simulink model "Pacemaker_Simulink"  (R2023a)
settings: Solver=FixedStepAuto  StartTime=0.0  StopTime=10.0  FixedStep=1e-3  RelTol=1e-3  EnableMultiTasking=on
undefined symbols (not defined in the file): A0, A1, D0, D1, D10, D11, D12, D13, D2, D3, D4, D5, D6, D7, D8, D9, magnitude, PTA0, PTA1, PTA2, PTB2, PTB23, PTB3, PTB9, PTC16, PTC17, PTC2, PTC3, PTC4, PTD0, PTD1, PTD2, PTD3
libraries: simulink x26, frdmk64flib x20, etargetslib x2, dspstat3 x1
settings Model: ExtModeTrigDuration=5  Creator=anshm  LastModifiedBy=anshm
settings OptimizationCC: EnhancedBackFolding=on  PassReuseOutputArgsAs=Individual arguments  ZeroExternalMemoryAtStartup=off  ZeroInternalMemoryAtStartup=off  MaxStackSize=64  OptimizeBlockOrder=speed  DifferentSizesBufferReuse=on  OptimizationCustomize=off  EfficientTunableParamExpr=on
settings DebuggingCC: ParameterTunabilityLossMsg=error
settings HardwareCC: ProdBitPerPointer=32  ProdBitPerSizeT=32  ProdBitPerPtrDiffT=32  ProdLargestAtomicInteger=Long  ProdLargestAtomicFloat=Double  ProdWordSize=32  ProdHWDeviceType=ARM Compatible->ARM Cortex
settings SFSimCC: MATLABDynamicMemAlloc=off
settings RTWCC: Description=Embedded Coder  SystemTargetFile=ert.tlc  HardwareBoard=NXP FRDM-K64F  TLCOptions="-aInlineSetEventsForThisBaseRateFcn=TLC_FALSE -aSuppressMultiTaskScheduler=TLC_FALSE  -aRateBasedStepFcn=0"  TemplateMakefile=ert_default_tmf  Toolchain=GNU Tools for ARM Embedded Processors
settings CodeAppCC: ForceParamTrailComments=on  IgnoreCustomStorageClasses=off  OperatorAnnotations=on  SimulinkDataObjDesc=on  SFDataObjDesc=on  InsertBlockDesc=on
settings ERTTargetCC: ExtModeTransport=4  ExtModeMexFile=sendToCommService

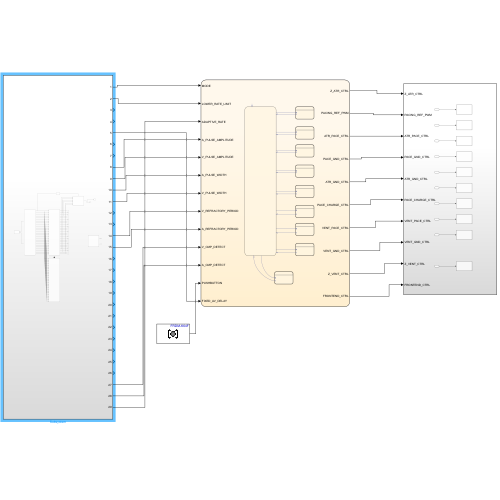
[thumbnail: Simulink's stored preview of the top-level diagram]
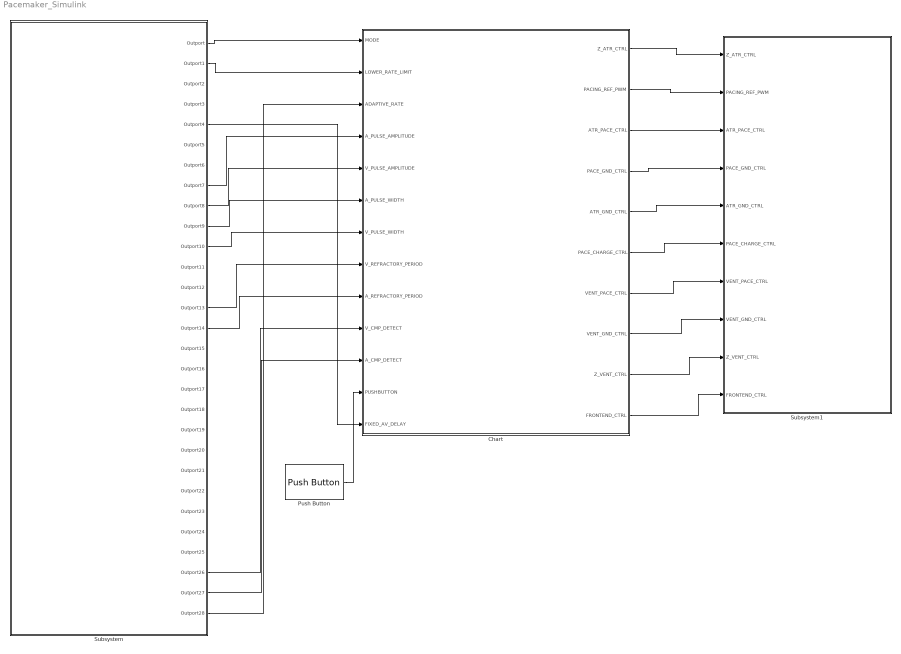
== system Pacemaker_Simulink ==
  Chart : Stateflow chart  TreatAsAtomicUnit=on
  Push Button : frdmk64flib/Push Button  Whichswitch=SW3  SampleTime1=-1
  Subsystem : Subsystem
  Subsystem1 : Subsystem
  wires:
  Chart/9(Z_VENT_CTRL) -> Subsystem1/9(Z_VENT_CTRL)
  Chart/8(VENT_GND_CTRL) -> Subsystem1/8(VENT_GND_CTRL)
  Chart/7(VENT_PACE_CTRL) -> Subsystem1/7(VENT_PACE_CTRL)
  Chart/6(PACE_CHARGE_CTRL) -> Subsystem1/6(PACE_CHARGE_CTRL)
  Chart/5(ATR_GND_CTRL) -> Subsystem1/5(ATR_GND_CTRL)
  Chart/4(PACE_GND_CTRL) -> Subsystem1/4(PACE_GND_CTRL)
  Chart/3(ATR_PACE_CTRL) -> Subsystem1/3(ATR_PACE_CTRL)
  Chart/2(PACING_REF_PWM) -> Subsystem1/2(PACING_REF_PWM)
  Chart/1(Z_ATR_CTRL) -> Subsystem1/1(Z_ATR_CTRL)
  Chart/10(FRONTEND_CTRL) -> Subsystem1/10(FRONTEND_CTRL)
  Subsystem/1(Outport) -> Chart/1(MODE)
  Subsystem/2(Outport1) -> Chart/2(LOWER_RATE_LIMIT)
  Subsystem/29(Outport28) -> Chart/3(ADAPTIVE_RATE)
  Subsystem/8(Outport7) -> Chart/4(A_PULSE_AMPLITUDE)
  Subsystem/9(Outport8) -> Chart/5(V_PULSE_AMPLITUDE)
  Subsystem/10(Outport9) -> Chart/6(A_PULSE_WIDTH)
  Subsystem/11(Outport10) -> Chart/7(V_PULSE_WIDTH)
  Subsystem/14(Outport13) -> Chart/8(V_REFRACTORY_PERIOD)
  Subsystem/15(Outport14) -> Chart/9(A_REFRACTORY_PERIOD)
  Subsystem/27(Outport26) -> Chart/10(V_CMP_DETECT)
  Subsystem/28(Outport27) -> Chart/11(A_CMP_DETECT)
  Push Button/1 -> Chart/12(PUSHBUTTON)
  Subsystem/5(Outport4) -> Chart/13(FIXED_AV_DELAY)

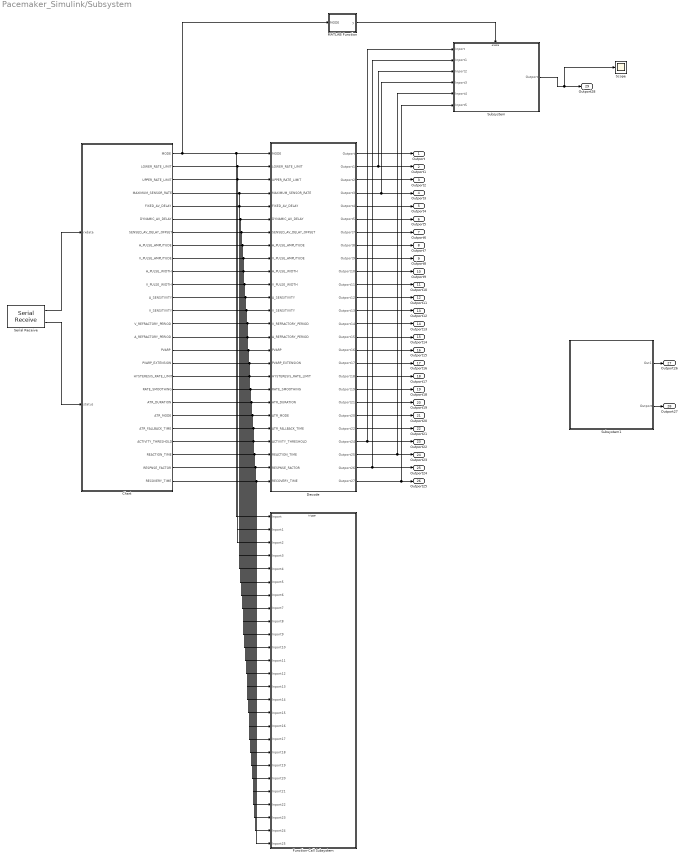
== system Pacemaker_Simulink/Subsystem ==
  Chart : Stateflow chart  TreatAsAtomicUnit=on
  Decode : Subsystem
  Function-Call Subsystem : Subsystem  TreatAsAtomicUnit=on
  MATLAB Function : MATLAB Function  TreatAsAtomicUnit=on
  Scope : Scope
  Serial Receive : frdmk64flib/Serial Receive  SCIModule=0  Baudrate=uint32(9600)  Parity=None  StopBits=1  HardwareFlowControl=None  ByteOrder=LittleEndian  DataType=uint8  DataLength=28  BlockingMode=off  OutputStatus=on  SampleTime=-1
  Subsystem : Subsystem
  Subsystem1 : Subsystem
  Outport : Outport
  Outport1 : Outport  Port=2
  Outport2 : Outport  Port=3
  Outport3 : Outport  Port=4
  Outport4 : Outport  Port=5
  Outport5 : Outport  Port=6
  Outport6 : Outport  Port=7
  Outport7 : Outport  Port=8
  Outport8 : Outport  Port=9
  Outport9 : Outport  Port=10
  Outport10 : Outport  Port=11
  Outport11 : Outport  Port=12
  Outport12 : Outport  Port=13
  Outport13 : Outport  Port=14
  Outport14 : Outport  Port=15
  Outport15 : Outport  Port=16
  Outport16 : Outport  Port=17
  Outport17 : Outport  Port=18
  Outport18 : Outport  Port=19
  Outport19 : Outport  Port=20
  Outport20 : Outport  Port=21
  Outport21 : Outport  Port=22
  Outport22 : Outport  Port=23
  Outport23 : Outport  Port=24
  Outport24 : Outport  Port=25
  Outport25 : Outport  Port=26
  Outport26 : Outport  Port=27
  Outport27 : Outport  Port=28
  Outport28 : Outport  Port=29
  wires:
  MATLAB Function/1(y) -> Subsystem/Enable
  Subsystem/1(Outport) -> Outport28/1, Scope/1
  Decode/18(Outport18) -> Outport17/1
  Decode/20(Outport21) -> Outport19/1
  Decode/14(Outport14) -> Outport13/1
  Serial Receive/2 -> Chart/2(status)
  Decode/19(Outport19) -> Outport18/1
  Decode/21(Outport20) -> Outport20/1
  Chart/9(V_PULSE_AMPLITUDE) -> Function-Call Subsystem/9(Inport8), Decode/9(V_PULSE_AMPLITUDE)
  Decode/12(Outport12) -> Outport11/1
  Chart/12(A_SENSITIVITY) -> Function-Call Subsystem/12(Inport11), Decode/12(A_SENSITIVITY)
  Decode/16(Outport16) -> Outport15/1
  Decode/15(Outport15) -> Outport14/1
  Decode/17(Outport17) -> Outport16/1
  Decode/13(Outport13) -> Outport12/1
  Chart/2(LOWER_RATE_LIMIT) -> Function-Call Subsystem/2(Inport1), Decode/2(LOWER_RATE_LIMIT)
  Chart/1(MODE) -> MATLAB Function/1(MODE), Function-Call Subsystem/1(Inport), Decode/1(MODE)
  Decode/10(Outport10) -> Outport9/1
  Chart/18(HYSTERESIS_RATE_LIMIT) -> Function-Call Subsystem/18(Inport17), Decode/18(HYSTERESIS_RATE_LIMIT)
  Decode/25(Outport26) -> Subsystem/2(Inport1), Outport24/1
  Decode/9(Outport9) -> Outport8/1
  Chart/20(ATR_DURATION) -> Function-Call Subsystem/20(Inport19), Decode/20(ATR_DURATION)
  Decode/11(Outport11) -> Outport10/1
  Decode/4(Outport3) -> Subsystem/4(Inport3), Outport3/1
  Decode/7(Outport7) -> Outport6/1
  Decode/8(Outport8) -> Outport7/1
  Chart/5(FIXED_AV_DELAY) -> Function-Call Subsystem/5(Inport4), Decode/5(FIXED_AV_DELAY)
  Chart/6(DYNAMIC_AV_DELAY) -> Function-Call Subsystem/6(Inport5), Decode/6(DYNAMIC_AV_DELAY)
  Decode/5(Outport4) -> Outport4/1
  Decode/3(Outport2) -> Outport2/1
  Decode/24(Outport25) -> Subsystem/5(Inport4), Outport23/1
  Chart/17(PVARP_EXTENSION) -> Function-Call Subsystem/17(Inport16), Decode/17(PVARP_EXTENSION)
  Chart/26(RECOVERY_TIME) -> Function-Call Subsystem/26(Inport25), Decode/26(RECOVERY_TIME)
  Decode/26(Outport27) -> Subsystem/6(Inport5), Outport25/1
  Chart/25(RESPNSE_FACTOR) -> Function-Call Subsystem/25(Inport24), Decode/25(RESPNSE_FACTOR)
  Chart/24(REACTION_TIME) -> Function-Call Subsystem/24(Inport23), Decode/24(REACTION_TIME)
  Chart/23(ACTIVITY_THRESHOLD) -> Function-Call Subsystem/23(Inport22), Decode/23(ACTIVITY_THRESHOLD)
  Chart/3(UPPER_RATE_LIMIT) -> Function-Call Subsystem/3(Inport2), Decode/3(UPPER_RATE_LIMIT)
  Chart/15(A_REFRACTORY_PERIOD) -> Function-Call Subsystem/15(Inport14), Decode/15(A_REFRACTORY_PERIOD)
  Chart/11(V_PULSE_WIDTH) -> Function-Call Subsystem/11(Inport10), Decode/11(V_PULSE_WIDTH)
  Chart/14(V_REFRACTORY_PERIOD) -> Function-Call Subsystem/14(Inport13), Decode/14(V_REFRACTORY_PERIOD)
  Chart/22(ATR_FALLBACK_TIME) -> Function-Call Subsystem/22(Inport21), Decode/22(ATR_FALLBACK_TIME)
  Chart/16(PVARP) -> Function-Call Subsystem/16(Inport15), Decode/16(PVARP)
  Chart/19(RATE_SMOOTHING) -> Function-Call Subsystem/19(Inport18), Decode/19(RATE_SMOOTHING)
  Decode/1(Outport) -> Outport/1
  Chart/13(V_SENSITIVITY) -> Function-Call Subsystem/13(Inport12), Decode/13(V_SENSITIVITY)
  Chart/21(ATR_MODE) -> Function-Call Subsystem/21(Inport20), Decode/21(ATR_MODE)
  Decode/2(Outport1) -> Subsystem/3(Inport2), Outport1/1
  Chart/4(MAXIMUM_SENSOR_RATE) -> Function-Call Subsystem/4(Inport3), Decode/4(MAXIMUM_SENSOR_RATE)
  Decode/6(Outport5) -> Outport5/1
  Decode/23(Outport24) -> Subsystem/1(Inport), Outport22/1
  Chart/8(A_PULSE_AMPLITUDE) -> Function-Call Subsystem/8(Inport7), Decode/8(A_PULSE_AMPLITUDE)
  Chart/7(SENSED_AV_DELAY_OFFSET) -> Function-Call Subsystem/7(Inport6), Decode/7(SENSED_AV_DELAY_OFFSET)
  Serial Receive/1 -> Chart/1(rxdata)
  Decode/22(Outport22) -> Outport21/1
  Chart/10(A_PULSE_WIDTH) -> Function-Call Subsystem/10(Inport9), Decode/10(A_PULSE_WIDTH)
  Subsystem1/2(Outport) -> Outport27/1
  Subsystem1/1(Out1) -> Outport26/1

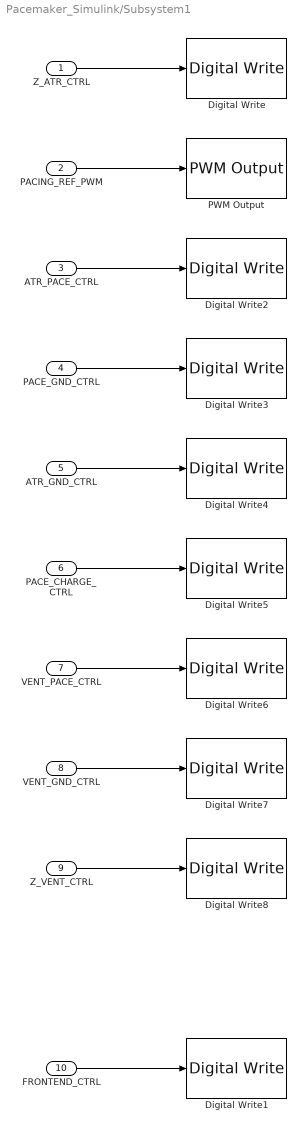
== system Pacemaker_Simulink/Subsystem1 ==
  Z_ATR_CTRL : Inport
  PACING_REF_PWM : Inport  Port=2
  ATR_PACE_CTRL : Inport  Port=3
  PACE_GND_CTRL : Inport  Port=4
  ATR_GND_CTRL : Inport  Port=5
  PACE_CHARGE_CTRL : Inport  Port=6
  VENT_PACE_CTRL : Inport  Port=7
  VENT_GND_CTRL : Inport  Port=8
  Z_VENT_CTRL : Inport  Port=9
  FRONTEND_CTRL : Inport  Port=10
  Digital Write : frdmk64flib/Digital Write  Whichpin=PTB23 (D4)
  Digital Write1 : frdmk64flib/Digital Write  Whichpin=PTD1 (D13)
  Digital Write2 : frdmk64flib/Digital Write  Whichpin=PTA0 (D8)
  Digital Write3 : frdmk64flib/Digital Write  Whichpin=PTD0 (D10)
  Digital Write4 : frdmk64flib/Digital Write  Whichpin=PTD2 (D11)
  Digital Write5 : frdmk64flib/Digital Write  Whichpin=PTB9 (D2)
  Digital Write6 : frdmk64flib/Digital Write  Whichpin=PTC4 (D9)
  Digital Write7 : frdmk64flib/Digital Write  Whichpin=PTD3 (D12)
  Digital Write8 : frdmk64flib/Digital Write  Whichpin=PTC3 (D7)
  PWM Output : frdmk64flib/PWM Output  Whichpin=PTA2 (D5)  InitialFrequency=2000  InitialDutyCycle=0
  wires:
  Z_ATR_CTRL/1 -> Digital Write/1
  ATR_GND_CTRL/1 -> Digital Write4/1
  PACE_CHARGE_CTRL/1 -> Digital Write5/1
  Z_VENT_CTRL/1 -> Digital Write8/1
  VENT_GND_CTRL/1 -> Digital Write7/1
  VENT_PACE_CTRL/1 -> Digital Write6/1
  PACING_REF_PWM/1 -> PWM Output/1
  ATR_PACE_CTRL/1 -> Digital Write2/1
  PACE_GND_CTRL/1 -> Digital Write3/1
  FRONTEND_CTRL/1 -> Digital Write1/1

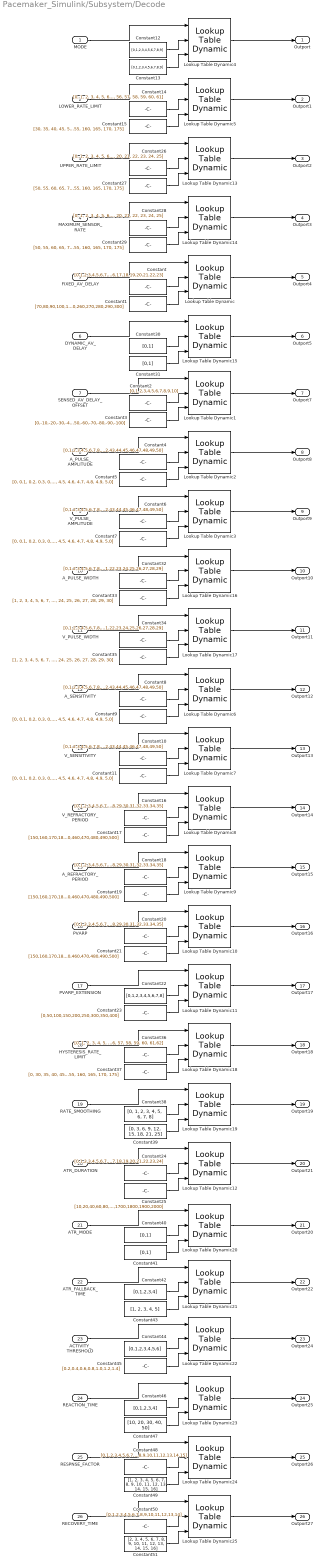
== system Pacemaker_Simulink/Subsystem/Decode ==
  MODE : Inport
  LOWER_RATE_LIMIT : Inport  Port=2
  UPPER_RATE_LIMIT : Inport  Port=3
  MAXIMUM_SENSOR_RATE : Inport  Port=4
  FIXED_AV_DELAY : Inport  Port=5
  DYNAMIC_AV_DELAY : Inport  Port=6
  SENSED_AV_DELAY_OFFSET : Inport  Port=7
  A_PULSE_AMPLITUDE : Inport  Port=8
  V_PULSE_AMPLITUDE : Inport  Port=9
  A_PULSE_WIDTH : Inport  Port=10
  V_PULSE_WIDTH : Inport  Port=11
  A_SENSITIVITY : Inport  Port=12
  V_SENSITIVITY : Inport  Port=13
  V_REFRACTORY_PERIOD : Inport  Port=14
  A_REFRACTORY_PERIOD : Inport  Port=15
  PVARP : Inport  Port=16
  PVARP_EXTENSION : Inport  Port=17
  HYSTERESIS_RATE_LIMIT : Inport  Port=18
  RATE_SMOOTHING : Inport  Port=19
  ATR_DURATION : Inport  Port=20
  ATR_MODE : Inport  Port=21
  ATR_FALLBACK_TIME : Inport  Port=22
  ACTIVITY_THRESHOLD : Inport  Port=23
  REACTION_TIME : Inport  Port=24
  RESPNSE_FACTOR : Inport  Port=25
  RECOVERY_TIME : Inport  Port=26
  Constant : Constant  Value=[0,1,2,3,4,5,6,7,8,9,10,11,12,13,14,15,16,17,18,19,20,21,22,23]
  Constant1 : Constant  Value=[70,80,90,100,110,120,130,140,150,160,170,180,190,200,210,220,230,240,250,260,270,280,290,300]
  Constant{4,6,8,10} (4 alike) : Constant  Value=[0,1,2,3,4,5,6,7,8,9,10,11,12,13,14,15,16,17,18,19,20,21,22,23,24,25,26,27,28,29,30,31,32,33,34,35,36,37,38,39,40,41,42,43,44,45,46,47,48,49,50]
  Constant{5,7,9,11} (4 alike) : Constant  Value=[0, 0.1, 0.2, 0.3, 0.4, 0.5, 0.6, 0.7, 0.8, 0.9, 1.0, 1.1, 1.2, 1.3, 1.4, 1.5, 1.6, 1.7, 1.8, 1.9, 2.0, 2.1, 2.2, 2.3, 2.4, 2.5, 2.6, 2.7, 2.8, 2.9, 3.0, 3.1, 3.2, 3.3, 3.4, 3.5, 3.6, 3.7, 3.8, 3.9, 4.0, 4.1, 4.2, 4.3, 4.4, 4.5, 4.6, 4.7, 4.8, 4.9, 5.0]
  Constant12 : Constant  Value=[0,1,2,3,4,5,6,7,8,9]
  Constant13 : Constant  Value=[0,1,2,3,4,5,6,7,8,9]
  Constant14 : Constant  Value=[0, 1, 2, 3, 4, 5, 6, 7, 8, 9, 10, 11, 12, 13, 14, 15, 16, 17, 18, 19, 20, 21, 22, 23, 24, 25, 26, 27, 28, 29, 30, 31, 32, 33, 34, 35, 36, 37, 38, 39, 40, 41, 42, 43, 44, 45, 46, 47, 48, 49, 50, 51, 52, 53, 54, 55, 56, 57, 58, 59, 60, 61]
  Constant15 : Constant  Value=[30, 35, 40, 45, 50, 51, 52, 53, 54, 55, 56, 57, 58, 59, 60, 61, 62, 63, 64, 65, 66, 67, 68, 69, 70, 71, 72, 73, 74, 75, 76, 77, 78, 79, 80, 81, 82, 83, 84, 85, 86, 87, 88, 89, 90, 95, 100, 105, 110, 115, 120, 125, 130, 135, 140, 145, 150, 155, 160, 165, 170, 175]
  Constant16 : Constant  Value=[0,1,2,3,4,5,6,7,8,9,10,11,12,13,14,15,16,17,18,19,20,21,22,23,24,25,26,27,28,29,30,31,32,33,34,35]
  Constant17 : Constant  Value=[150,160,170,180,190,200,210,220,230,240,250,260,270,280,290,300,310,320,330,340,350,360,370,380,390,400,410,420,430,440,450,460,470,480,490,500]
  Constant18 : Constant  Value=[0,1,2,3,4,5,6,7,8,9,10,11,12,13,14,15,16,17,18,19,20,21,22,23,24,25,26,27,28,29,30,31,32,33,34,35]
  Constant19 : Constant  Value=[150,160,170,180,190,200,210,220,230,240,250,260,270,280,290,300,310,320,330,340,350,360,370,380,390,400,410,420,430,440,450,460,470,480,490,500]
  Constant2 : Constant  Value=[0,1,2,3,4,5,6,7,8,9,10]
  Constant20 : Constant  Value=[0,1,2,3,4,5,6,7,8,9,10,11,12,13,14,15,16,17,18,19,20,21,22,23,24,25,26,27,28,29,30,31,32,33,34,35]
  Constant21 : Constant  Value=[150,160,170,180,190,200,210,220,230,240,250,260,270,280,290,300,310,320,330,340,350,360,370,380,390,400,410,420,430,440,450,460,470,480,490,500]
  Constant22 : Constant  Value=[0,1,2,3,4,5,6,7,8]
  Constant23 : Constant  Value=[0,50,100,150,200,250,300,350,400]
  Constant24 : Constant  Value=[0,1,2,3,4,5,6,7,8,9,10,11,12,13,14,15,16,17,18,19,20,21,22,23,24]
  Constant25 : Constant  Value=[10,20,40,60,80,100,200,300,400,500,600,700,800,900,1000,1100,1200,1300,1400,1500,1600,1700,1800,1900,2000]
  Constant26 : Constant  Value=[0, 1, 2, 3, 4, 5, 6, 7, 8, 9, 10, 11, 12, 13, 14, 15, 16, 17, 18, 19, 20, 21, 22, 23, 24, 25]
  Constant27 : Constant  Value=[50, 55, 60, 65, 70, 75, 80, 85, 90, 95, 100, 105, 110, 115, 120, 125, 130, 135, 140, 145, 150, 155, 160, 165, 170, 175]
  Constant28 : Constant  Value=[0, 1, 2, 3, 4, 5, 6, 7, 8, 9, 10, 11, 12, 13, 14, 15, 16, 17, 18, 19, 20, 21, 22, 23, 24, 25]
  Constant29 : Constant  Value=[50, 55, 60, 65, 70, 75, 80, 85, 90, 95, 100, 105, 110, 115, 120, 125, 130, 135, 140, 145, 150, 155, 160, 165, 170, 175]
  Constant3 : Constant  Value=[0,-10,-20,-30,-40,-50,-60,-70,-80,-90,-100]
  Constant{30..31,40..41} (4 alike) : Constant  Value=[0,1]
  Constant32 : Constant  Value=[0,1,2,3,4,5,6,7,8,9,10,11,12,13,14,15,16,17,18,19,20,21,22,23,24,25,26,27,28,29]
  Constant33 : Constant  Value=[1, 2, 3, 4, 5, 6, 7, 8, 9, 10, 11, 12, 13, 14, 15, 16, 17, 18, 19, 20, 21, 22, 23, 24, 25, 26, 27, 28, 29, 30]
  Constant34 : Constant  Value=[0,1,2,3,4,5,6,7,8,9,10,11,12,13,14,15,16,17,18,19,20,21,22,23,24,25,26,27,28,29]
  Constant35 : Constant  Value=[1, 2, 3, 4, 5, 6, 7, 8, 9, 10, 11, 12, 13, 14, 15, 16, 17, 18, 19, 20, 21, 22, 23, 24, 25, 26, 27, 28, 29, 30]
  Constant36 : Constant  Value=[0, 1, 2, 3, 4, 5, 6, 7, 8, 9, 10, 11, 12, 13, 14, 15, 16, 17, 18, 19, 20, 21, 22, 23, 24, 25, 26, 27, 28, 29, 30, 31, 32, 33, 34, 35, 36, 37, 38, 39, 40, 41, 42, 43, 44, 45, 46, 47, 48, 49, 50, 51, 52, 53, 54, 55, 56, 57, 58, 59, 60, 61,62]
  Constant37 : Constant  Value=[0, 30, 35, 40, 45, 50, 51, 52, 53, 54, 55, 56, 57, 58, 59, 60, 61, 62, 63, 64, 65, 66, 67, 68, 69, 70, 71, 72, 73, 74, 75, 76, 77, 78, 79, 80, 81, 82, 83, 84, 85, 86, 87, 88, 89, 90, 95, 100, 105, 110, 115, 120, 125, 130, 135, 140, 145, 150, 155, 160, 165, 170, 175]
  Constant38 : Constant  Value=[0, 1, 2, 3, 4, 5, 6, 7, 8]
  Constant39 : Constant  Value=[0, 3, 6, 9, 12, 15, 18, 21, 25]
  Constant42 : Constant  Value=[0,1,2,3,4]
  Constant43 : Constant  Value=[1, 2, 3, 4, 5]
  Constant44 : Constant  Value=[0,1,2,3,4,5,6]
  Constant45 : Constant  Value=[0.2,0.4,0.6,0.8,1.0,1.2,1.4]
  Constant46 : Constant  Value=[0,1,2,3,4]
  Constant47 : Constant  Value=[10, 20, 30, 40, 50]
  Constant48 : Constant  Value=[0,1,2,3,4,5,6,7,8,9,10,11,12,13,14,15]
  Constant49 : Constant  Value=[1, 2, 3, 4, 5, 6, 7, 8, 9, 10, 11, 12, 13, 14, 15, 16]
  Constant50 : Constant  Value=[0,1,2,3,4,5,6,7,8,9,10,11,12,13,14]
  Constant51 : Constant  Value=[2, 3, 4, 5, 6, 7, 8, 9, 10, 11, 12, 13, 14, 15, 16]
  Lookup Table Dynamic{,1..25} (26 alike) : simulink/Lookup Tables/Lookup Table Dynamic  LookUpMeth=Interpolation-Use End Values  OutDataType=fixdt('double')  OutScaling=[]  OutputDataTypeScalingMode=Specify via dialog  OutDataTypeStr=double  DoSatur=off
  Outport : Outport
  Outport1 : Outport  Port=2
  Outport2 : Outport  Port=3
  Outport3 : Outport  Port=4
  Outport4 : Outport  Port=5
  Outport5 : Outport  Port=6
  Outport7 : Outport  Port=7
  Outport8 : Outport  Port=8
  Outport9 : Outport  Port=9
  Outport10 : Outport  Port=10
  Outport11 : Outport  Port=11
  Outport12 : Outport  Port=12
  Outport13 : Outport  Port=13
  Outport14 : Outport  Port=14
  Outport15 : Outport  Port=15
  Outport16 : Outport  Port=16
  Outport17 : Outport  Port=17
  Outport18 : Outport  Port=18
  Outport19 : Outport  Port=19
  Outport21 : Outport  Port=20
  Outport20 : Outport  Port=21
  Outport22 : Outport  Port=22
  Outport24 : Outport  Port=23
  Outport25 : Outport  Port=24
  Outport26 : Outport  Port=25
  Outport27 : Outport  Port=26
  wires:
  Lookup Table Dynamic/1 -> Outport4/1
  FIXED_AV_DELAY/1 -> Lookup Table Dynamic/1
  Constant/1 -> Lookup Table Dynamic/2
  Constant1/1 -> Lookup Table Dynamic/3
  Lookup Table Dynamic1/1 -> Outport7/1
  SENSED_AV_DELAY_OFFSET/1 -> Lookup Table Dynamic1/1
  Constant3/1 -> Lookup Table Dynamic1/3
  Constant2/1 -> Lookup Table Dynamic1/2
  Constant5/1 -> Lookup Table Dynamic2/3
  Constant4/1 -> Lookup Table Dynamic2/2
  A_PULSE_AMPLITUDE/1 -> Lookup Table Dynamic2/1
  Lookup Table Dynamic2/1 -> Outport8/1
  Lookup Table Dynamic3/1 -> Outport9/1
  Constant6/1 -> Lookup Table Dynamic3/2
  Constant7/1 -> Lookup Table Dynamic3/3
  V_PULSE_AMPLITUDE/1 -> Lookup Table Dynamic3/1
  Constant8/1 -> Lookup Table Dynamic6/2
  Lookup Table Dynamic6/1 -> Outport12/1
  A_SENSITIVITY/1 -> Lookup Table Dynamic6/1
  Constant9/1 -> Lookup Table Dynamic6/3
  Lookup Table Dynamic7/1 -> Outport13/1
  Constant11/1 -> Lookup Table Dynamic7/3
  Constant10/1 -> Lookup Table Dynamic7/2
  V_SENSITIVITY/1 -> Lookup Table Dynamic7/1
  Constant16/1 -> Lookup Table Dynamic8/2
  Constant17/1 -> Lookup Table Dynamic8/3
  V_REFRACTORY_PERIOD/1 -> Lookup Table Dynamic8/1
  Lookup Table Dynamic8/1 -> Outport14/1
  A_REFRACTORY_PERIOD/1 -> Lookup Table Dynamic9/1
  Constant18/1 -> Lookup Table Dynamic9/2
  Lookup Table Dynamic9/1 -> Outport15/1
  Constant19/1 -> Lookup Table Dynamic9/3
  PVARP/1 -> Lookup Table Dynamic10/1
  Constant20/1 -> Lookup Table Dynamic10/2
  Constant21/1 -> Lookup Table Dynamic10/3
  Lookup Table Dynamic10/1 -> Outport16/1
  PVARP_EXTENSION/1 -> Lookup Table Dynamic11/1
  Constant22/1 -> Lookup Table Dynamic11/2
  Constant23/1 -> Lookup Table Dynamic11/3
  ATR_DURATION/1 -> Lookup Table Dynamic12/1
  Constant24/1 -> Lookup Table Dynamic12/2
  Constant25/1 -> Lookup Table Dynamic12/3
  Lookup Table Dynamic12/1 -> Outport21/1
  MODE/1 -> Lookup Table Dynamic4/1
  Lookup Table Dynamic4/1 -> Outport/1
  Constant12/1 -> Lookup Table Dynamic4/2
  Constant13/1 -> Lookup Table Dynamic4/3
  LOWER_RATE_LIMIT/1 -> Lookup Table Dynamic5/1
  Lookup Table Dynamic5/1 -> Outport1/1
  Constant15/1 -> Lookup Table Dynamic5/3
  Constant14/1 -> Lookup Table Dynamic5/2
  Constant26/1 -> Lookup Table Dynamic13/2
  UPPER_RATE_LIMIT/1 -> Lookup Table Dynamic13/1
  Constant27/1 -> Lookup Table Dynamic13/3
  Lookup Table Dynamic13/1 -> Outport2/1
  Constant29/1 -> Lookup Table Dynamic14/3
  Constant28/1 -> Lookup Table Dynamic14/2
  MAXIMUM_SENSOR_RATE/1 -> Lookup Table Dynamic14/1
  Lookup Table Dynamic14/1 -> Outport3/1
  DYNAMIC_AV_DELAY/1 -> Lookup Table Dynamic15/1
  Constant30/1 -> Lookup Table Dynamic15/2
  Constant31/1 -> Lookup Table Dynamic15/3
  Lookup Table Dynamic15/1 -> Outport5/1
  Constant32/1 -> Lookup Table Dynamic16/2
  Constant33/1 -> Lookup Table Dynamic16/3
  A_PULSE_WIDTH/1 -> Lookup Table Dynamic16/1
  Lookup Table Dynamic16/1 -> Outport10/1
  V_PULSE_WIDTH/1 -> Lookup Table Dynamic17/1
  Constant35/1 -> Lookup Table Dynamic17/3
  Constant34/1 -> Lookup Table Dynamic17/2
  Lookup Table Dynamic17/1 -> Outport11/1
  Constant37/1 -> Lookup Table Dynamic18/3
  Constant36/1 -> Lookup Table Dynamic18/2
  HYSTERESIS_RATE_LIMIT/1 -> Lookup Table Dynamic18/1
  Lookup Table Dynamic11/1 -> Outport17/1
  Lookup Table Dynamic18/1 -> Outport18/1
  RATE_SMOOTHING/1 -> Lookup Table Dynamic19/1
  Constant39/1 -> Lookup Table Dynamic19/3
  Constant38/1 -> Lookup Table Dynamic19/2
  Lookup Table Dynamic19/1 -> Outport19/1
  Constant41/1 -> Lookup Table Dynamic20/3
  Constant40/1 -> Lookup Table Dynamic20/2
  ATR_MODE/1 -> Lookup Table Dynamic20/1
  Lookup Table Dynamic20/1 -> Outport20/1
  ATR_FALLBACK_TIME/1 -> Lookup Table Dynamic21/1
  Constant43/1 -> Lookup Table Dynamic21/3
  Constant42/1 -> Lookup Table Dynamic21/2
  Lookup Table Dynamic21/1 -> Outport22/1
  ACTIVITY_THRESHOLD/1 -> Lookup Table Dynamic22/1
  Constant44/1 -> Lookup Table Dynamic22/2
  Constant45/1 -> Lookup Table Dynamic22/3
  Lookup Table Dynamic22/1 -> Outport24/1
  Constant47/1 -> Lookup Table Dynamic23/3
  Constant46/1 -> Lookup Table Dynamic23/2
  REACTION_TIME/1 -> Lookup Table Dynamic23/1
  Lookup Table Dynamic23/1 -> Outport25/1
  RESPNSE_FACTOR/1 -> Lookup Table Dynamic24/1
  Constant48/1 -> Lookup Table Dynamic24/2
  Constant49/1 -> Lookup Table Dynamic24/3
  Lookup Table Dynamic24/1 -> Outport26/1
  RECOVERY_TIME/1 -> Lookup Table Dynamic25/1
  Constant50/1 -> Lookup Table Dynamic25/2
  Constant51/1 -> Lookup Table Dynamic25/3
  Lookup Table Dynamic25/1 -> Outport27/1

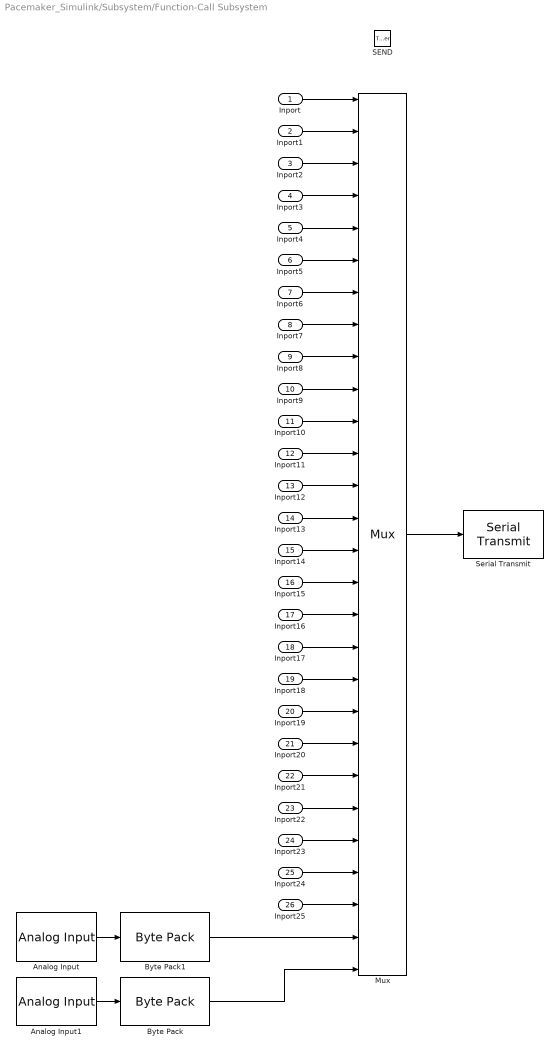
== system Pacemaker_Simulink/Subsystem/Function-Call Subsystem ==
  Inport : Inport
  Inport1 : Inport  Port=2
  Inport2 : Inport  Port=3
  Inport3 : Inport  Port=4
  Inport4 : Inport  Port=5
  Inport5 : Inport  Port=6
  Inport6 : Inport  Port=7
  Inport7 : Inport  Port=8
  Inport8 : Inport  Port=9
  Inport9 : Inport  Port=10
  Inport10 : Inport  Port=11
  Inport11 : Inport  Port=12
  Inport12 : Inport  Port=13
  Inport13 : Inport  Port=14
  Inport14 : Inport  Port=15
  Inport15 : Inport  Port=16
  Inport16 : Inport  Port=17
  Inport17 : Inport  Port=18
  Inport18 : Inport  Port=19
  Inport19 : Inport  Port=20
  Inport20 : Inport  Port=21
  Inport21 : Inport  Port=22
  Inport22 : Inport  Port=23
  Inport23 : Inport  Port=24
  Inport24 : Inport  Port=25
  Inport25 : Inport  Port=26
  SEND : TriggerPort  TriggerType=function-call  IsSimulinkFunction=on  FunctionName=SEND  VariantControl=(inherit)
  Analog Input : frdmk64flib/Analog Input  Whichpin=PTB3 (A1)  SampleTime=-1
  Analog Input1 : frdmk64flib/Analog Input  Whichpin=PTB2 (A0)  SampleTime=-1
  Byte Pack : etargetslib/Byte Pack  datatypes={'double'}  byteAlign=1
  Byte Pack1 : etargetslib/Byte Pack  datatypes={'double'}  byteAlign=1
  Mux : Mux  Inputs=28
  Serial Transmit : frdmk64flib/Serial Transmit  SCIModule=0  Baudrate=uint32(9600)  Parity=None  StopBits=1  HardwareFlowControl=None  ByteOrder=LittleEndian  BlockingMode=on  OutputStatus=off
  wires:
  Mux/1 -> Serial Transmit/1
  Inport/1 -> Mux/1
  Inport1/1 -> Mux/2
  Inport2/1 -> Mux/3
  Inport3/1 -> Mux/4
  Inport4/1 -> Mux/5
  Inport5/1 -> Mux/6
  Inport6/1 -> Mux/7
  Inport7/1 -> Mux/8
  Inport8/1 -> Mux/9
  Inport9/1 -> Mux/10
  Inport10/1 -> Mux/11
  Inport11/1 -> Mux/12
  Inport12/1 -> Mux/13
  Inport13/1 -> Mux/14
  Inport14/1 -> Mux/15
  Inport15/1 -> Mux/16
  Inport16/1 -> Mux/17
  Inport17/1 -> Mux/18
  Inport18/1 -> Mux/19
  Inport19/1 -> Mux/20
  Inport20/1 -> Mux/21
  Inport21/1 -> Mux/22
  Inport22/1 -> Mux/23
  Inport23/1 -> Mux/24
  Inport24/1 -> Mux/25
  Inport25/1 -> Mux/26
  Analog Input1/1 -> Byte Pack/1
  Analog Input/1 -> Byte Pack1/1
  Byte Pack1/1 -> Mux/27
  Byte Pack/1 -> Mux/28

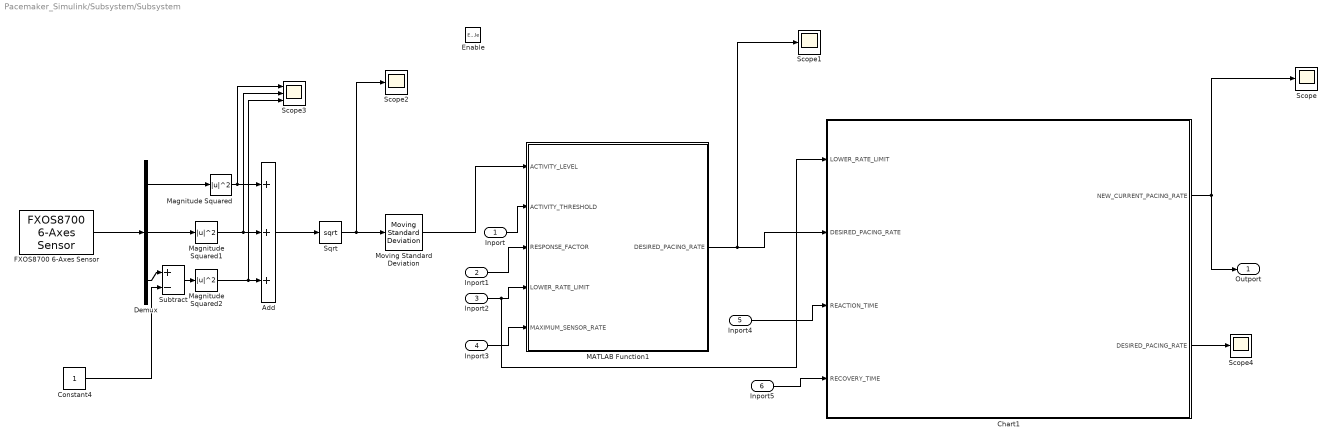
== system Pacemaker_Simulink/Subsystem/Subsystem ==
  Inport : Inport
  Inport1 : Inport  Port=2
  Inport2 : Inport  Port=3
  Inport3 : Inport  Port=4
  Inport4 : Inport  Port=5
  Inport5 : Inport  Port=6
  Enable : EnablePort
  Add : Sum  Inputs=+++
  Chart1 : Stateflow chart  TreatAsAtomicUnit=on
  Constant4 : Constant
  Demux : Demux  Outputs=3
  FXOS8700 6-Axes Sensor : frdmk64flib/FXOS8700 6-Axes Sensor  Activesensor=Accelerometer only  ODR=200Hz  HybridODR=400Hz  Accelfullrange=-4g to +4g  SampleTime=-1
  MATLAB Function1 : MATLAB Function  TreatAsAtomicUnit=on
  Magnitude Squared : Math  Operator=magnitude^2
  Magnitude Squared1 : Math  Operator=magnitude^2
  Magnitude Squared2 : Math  Operator=magnitude^2
  Moving Standard Deviation : dspstat3/Moving Standard Deviation  Method=Sliding window  ForgettingFactorPort=off  SpecifyWindowLength=on  WindowLength=150  OverlapLength=149  AllowArbitraryInputLength=off  ForgettingFactor=0.9  SimulateUsing=Code generation
  Scope{,1..2,4} (4 alike) : Scope
  Scope3 : Scope  NumInputPorts=3
  Sqrt : Sqrt
  Subtract : Sum  Inputs=+-
  Outport : Outport
  wires:
  Add/1 -> Sqrt/1
  Magnitude Squared2/1 -> Scope3/3, Add/3
  Demux/2 -> Magnitude Squared1/1
  Sqrt/1 -> Moving Standard Deviation/1, Scope2/1
  Demux/1 -> Magnitude Squared/1
  Magnitude Squared/1 -> Scope3/1, Add/1
  Constant4/1 -> Subtract/2
  Magnitude Squared1/1 -> Scope3/2, Add/2
  FXOS8700 6-Axes Sensor/1 -> Demux/1
  Demux/3 -> Subtract/1
  Subtract/1 -> Magnitude Squared2/1
  Chart1/1(NEW_CURRENT_PACING_RATE) -> Outport/1, Scope/1
  Moving Standard Deviation/1 -> MATLAB Function1/1(ACTIVITY_LEVEL)
  Inport/1 -> MATLAB Function1/2(ACTIVITY_THRESHOLD)
  Inport1/1 -> MATLAB Function1/3(RESPONSE_FACTOR)
  Inport2/1 -> Chart1/1(LOWER_RATE_LIMIT), MATLAB Function1/4(LOWER_RATE_LIMIT)
  Inport3/1 -> MATLAB Function1/5(MAXIMUM_SENSOR_RATE)
  MATLAB Function1/1(DESIRED_PACING_RATE) -> Scope1/1, Chart1/2("DESIRED_PACING_RATE ")
  Inport4/1 -> Chart1/3(REACTION_TIME)
  Inport5/1 -> Chart1/4(RECOVERY_TIME)
  Chart1/2(DESIRED_PACING_RATE) -> Scope4/1

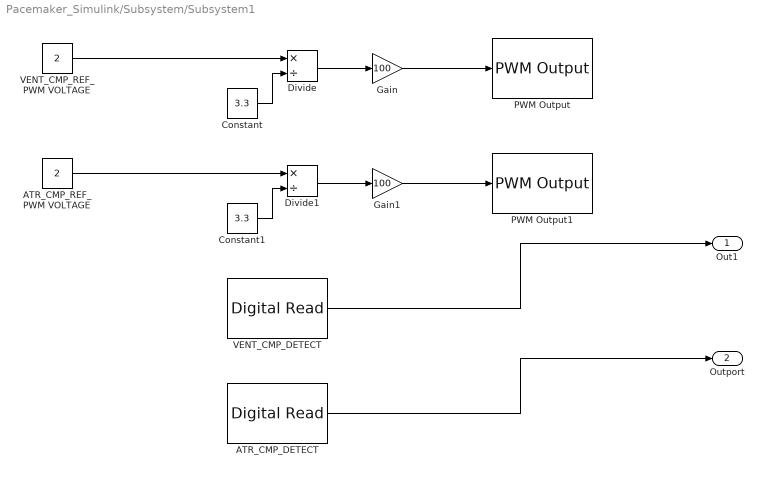
== system Pacemaker_Simulink/Subsystem/Subsystem1 ==
  ATR_CMP_DETECT : frdmk64flib/Digital Read  Whichpin=PTC16 (D0)  SampleTime=-1
  ATR_CMP_REF_PWM VOLTAGE : Constant  Value=2
  Constant : Constant  Value=3.3
  Constant1 : Constant  Value=3.3
  Divide : Product  Inputs=*/
  Divide1 : Product  Inputs=*/
  Gain : Gain  Gain=100
  Gain1 : Gain  Gain=100
  PWM Output : frdmk64flib/PWM Output  Whichpin=PTA1 (D3)  InitialFrequency=2000  InitialDutyCycle=0
  PWM Output1 : frdmk64flib/PWM Output  Whichpin=PTC2 (D6)  InitialFrequency=2000  InitialDutyCycle=0
  VENT_CMP_DETECT : frdmk64flib/Digital Read  Whichpin=PTC17 (D1)  SampleTime=-1
  VENT_CMP_REF_PWM VOLTAGE : Constant  Value=2
  Out1 : Outport
  Outport : Outport  Port=2
  wires:
  Gain1/1 -> PWM Output1/1
  VENT_CMP_DETECT/1 -> Out1/1
  VENT_CMP_REF_PWM VOLTAGE/1 -> Divide/1
  Constant/1 -> Divide/2
  ATR_CMP_DETECT/1 -> Outport/1
  Divide/1 -> Gain/1
  ATR_CMP_REF_PWM VOLTAGE/1 -> Divide1/1
  Divide1/1 -> Gain1/1
  Gain/1 -> PWM Output/1
  Constant1/1 -> Divide1/2

== stateflow chart Pacemaker_Simulink/Subsystem/Chart ==
  settings: executeAtInitialization=1
  state SET_PARAM
    entry:
    MODE = rxdata(3)
    LOWER_RATE_LIMIT = rxdata(4)
    UPPER_RATE_LIMIT = rxdata(5)
    MAXIMUM_SENSOR_RATE = rxdata(6)
    FIXED_AV_DELAY = rxdata(7)
    DYNAMIC_AV_DELAY = rxdata(8)
    SENSED_AV_DELAY_OFFSET = rxdata(9)
    A_PULSE_AMPLITUDE = rxdata(10)
    V_PULSE_AMPLITUDE = rxdata(11)
    A_PULSE_WIDTH = rxdata(12)
    V_PULSE_WIDTH = rxdata(13)
    A_SENSITIVITY = rxdata(14)
    V_SENSITIVITY = rxdata(15)
    V_REFRACTORY_PERIOD = rxdata(16)
    A_REFRACTORY_PERIOD = rxdata(17)
    PVARP = rxdata(18)
    PVARP_EXTENSION = rxdata(19)
    HYSTERESIS_RATE_LIMIT = rxdata(20)
    RATE_SMOOTHING = rxdata(21)
    ATR_DURATION = rxdata(22)
    ATR_MODE = rxdata(23)
    ATR_FALLBACK_TIME = rxdata(24)
    ACTIVITY_THRESHOLD = rxdata(25)
    REACTION_TIME = rxdata(26)
    RESPNSE_FACTOR = rxdata(27)
    RECOVERY_TIME = rxdata(28)
  state INITIAL
    entry:
    MODE = 9
    LOWER_RATE_LIMIT = 14
    UPPER_RATE_LIMIT = 14
    MAXIMUM_SENSOR_RATE = 14
    FIXED_AV_DELAY = 8
    DYNAMIC_AV_DELAY = 0
    SENSED_AV_DELAY_OFFSET = 0
    A_PULSE_AMPLITUDE = 29
    V_PULSE_AMPLITUDE = 29
    A_PULSE_WIDTH = 4
    V_PULSE_WIDTH = 4
    A_SENSITIVITY = 2
    V_SENSITIVITY = 6
    V_REFRACTORY_PERIOD = 16
    A_REFRACTORY_PERIOD = 9
    PVARP = 9
    PVARP_EXTENSION = 0
    HYSTERESIS_RATE_LIMIT = 0
    RATE_SMOOTHING = 0
    ATR_DURATION = 1
    ATR_MODE = 0
    ATR_FALLBACK_TIME = 0
    ACTIVITY_THRESHOLD = 0
    REACTION_TIME = 0
    RESPNSE_FACTOR = 15
    RECOVERY_TIME = 0
  state STANDBY
  state ECHO_PARAM
    entry:
    SEND();
  (default) -> INITIAL
  SET_PARAM -> STANDBY
  (junction 34) -> SET_PARAM [order 1] : [rxdata(2) == hex2dec('55')]
  (junction 33) -> STANDBY [order 2]
  INITIAL -> STANDBY
  (junction 33) -> (junction 34) [order 1] : [rxdata(1) == hex2dec('16')]
  STANDBY -> (junction 33) : [status == 0]
  (junction 34) -> ECHO_PARAM [order 2] : [rxdata(2) == hex2dec('22')]
  ECHO_PARAM -> STANDBY
  data: MODE output uint8; LOWER_RATE_LIMIT output uint8; UPPER_RATE_LIMIT output uint8; MAXIMUM_SENSOR_RATE output uint8; FIXED_AV_DELAY output uint8; DYNAMIC_AV_DELAY output uint8; SENSED_AV_DELAY_OFFSET output uint8; A_PULSE_AMPLITUDE output uint8; V_PULSE_AMPLITUDE output uint8; A_PULSE_WIDTH output uint8; V_PULSE_WIDTH output uint8; A_SENSITIVITY output uint8; V_SENSITIVITY output uint8; V_REFRACTORY_PERIOD output uint8; A_REFRACTORY_PERIOD output uint8; PVARP output uint8; PVARP_EXTENSION output uint8; HYSTERESIS_RATE_LIMIT output uint8; RATE_SMOOTHING output uint8; ATR_DURATION output uint8; ATR_MODE output uint8; ATR_FALLBACK_TIME output uint8; ACTIVITY_THRESHOLD output uint8; REACTION_TIME output uint8; RESPNSE_FACTOR output uint8; RECOVERY_TIME output uint8; rxdata input uint8; status input uint8; EG local

== stateflow chart Pacemaker_Simulink/Subsystem/Subsystem/Chart1 ==
  state INITIAL
    entry:
    NEW_CURRENT_PACING_RATE = LOWER_RATE_LIMIT;
  state STANDBY
    entry:
    RISE = abs(DESIRED_PACING_RATE - NEW_CURRENT_PACING_RATE)/(REACTION_TIME*1);
    FALL = abs(DESIRED_PACING_RATE - NEW_CURRENT_PACING_RATE)/(RECOVERY_TIME*1);
    NEW_CURRENT_PACING_RATE = NEW_CURRENT_PACING_RATE;
    DESIRED_PACING_RATE = DESIRED_PACING_RATE;
  state RISE1
    entry:
    NEW_CURRENT_PACING_RATE = NEW_CURRENT_PACING_RATE - FALL;
  state RISE
    entry:
    NEW_CURRENT_PACING_RATE = NEW_CURRENT_PACING_RATE + RISE;
  (default) -> INITIAL
  INITIAL -> STANDBY
  STANDBY -> RISE [order 1] : [NEW_CURRENT_PACING_RATE < DESIRED_PACING_RATE]
  STANDBY -> RISE1 [order 2] : [NEW_CURRENT_PACING_RATE > DESIRED_PACING_RATE]
  RISE -> STANDBY : [after(1000,msec)]
  RISE1 -> STANDBY : [after(1000,msec)]
  data: NEW_CURRENT_PACING_RATE output; LOWER_RATE_LIMIT input; DESIRED_PACING_RATE input; REACTION_TIME input; RECOVERY_TIME input; FALL local; RISE local; DESIRED_PACING_RATE output

== stateflow chart Pacemaker_Simulink/Chart ==
  state OFF
    entry:
    FRONTEND_CTRL = 1
  state AOO
    state State_1
      entry:
      %Charging C22
      ATR_PACE_CTRL = 0;
      VENT_PACE_CTRL = 0;
      PACING_REF_PWM = (A_PULSE_AMPLITUDE/5)*100;
      PACE_CHARGE_CTRL = 1;
      %Discharging Blocking Capacitor
      PACE_GND_CTRL = 1
      Z_ATR_CTRL = 0
      Z_VENT_CTRL = 0
      ATR_GND_CTRL = 1
      VENT_GND_CTRL = 0
    state State_2
      entry:
      %Atrium Pacing
      PACE_CHARGE_CTRL = 0
      PACE_GND_CTRL = 1
      ATR_PACE_CTRL = 1
      ATR_GND_CTRL = 0
      Z_ATR_CTRL = 0
      Z_VENT_CTRL = 0
      VENT_GND_CTRL = 0
      VENT_PACE_CTRL = 0
    AOO.State_1 -> AOO.State_2 [order 2] : [after((60000/LOWER_RATE_LIMIT) - A_PULSE_WIDTH,msec)] % (60000msec/min) / (pulse/min) = msec / 1 pulse
    AOO.State_2 -> AOO.State_1 : [after(A_PULSE_WIDTH, msec)]
  state VOO
    state State_1
      entry:
      %Charging C22
      ATR_PACE_CTRL = 0;
      VENT_PACE_CTRL = 0;
      PACING_REF_PWM = (V_PULSE_AMPLITUDE/5) * 100;
      PACE_CHARGE_CTRL = 1;
      %Discharging Blocking Capacitor
      PACE_GND_CTRL = 1
      Z_ATR_CTRL = 0
      Z_VENT_CTRL = 0
      ATR_GND_CTRL = 0
      VENT_GND_CTRL = 1
    state State_2
      entry:
      %Ventricle Pacing
      PACE_CHARGE_CTRL = 0
      PACE_GND_CTRL = 1
      ATR_PACE_CTRL = 0
      ATR_GND_CTRL = 0
      Z_ATR_CTRL = 0
      Z_VENT_CTRL = 0
      VENT_GND_CTRL = 0
      VENT_PACE_CTRL = 1
    VOO.State_1 -> VOO.State_2 [order 1] : [after((60000/LOWER_RATE_LIMIT) - V_PULSE_WIDTH,msec)] % (60000msec/min) / (pulse/min) = msec / 1 pulse
    VOO.State_2 -> VOO.State_1 : [after(V_PULSE_WIDTH, msec)]
  state AAI
    state State_1
      entry:
      FRONTEND_CTRL = 1
      %Charging C22
      ATR_PACE_CTRL = 0;
      VENT_PACE_CTRL = 0;
      PACING_REF_PWM = (A_PULSE_AMPLITUDE/5)*100;
      PACE_CHARGE_CTRL = 1;
      %Discharging Blocking Capacitor
      PACE_GND_CTRL = 1
      Z_ATR_CTRL = 0
      Z_VENT_CTRL = 0
      ATR_GND_CTRL = 1
      VENT_GND_CTRL = 0
    state State_2
      entry:
      %Atrium Pacing
      PACE_CHARGE_CTRL = 0
      PACE_GND_CTRL = 1
      ATR_PACE_CTRL = 1
      ATR_GND_CTRL = 0
      Z_ATR_CTRL = 0
      Z_VENT_CTRL = 0
      VENT_GND_CTRL = 0
      VENT_PACE_CTRL = 0
    state State_3
      entry:
      %Charging C22
      ATR_PACE_CTRL = 0;
      VENT_PACE_CTRL = 0;
      PACING_REF_PWM = (A_PULSE_AMPLITUDE/5)*100;
      PACE_CHARGE_CTRL = 1;
      %Discharging Blocking Capacitor
      PACE_GND_CTRL = 1
      Z_ATR_CTRL = 0
      Z_VENT_CTRL = 0
      ATR_GND_CTRL = 1
      VENT_GND_CTRL = 0
    AAI.State_1 -> AAI.State_2 [order 2] : after(((60000/LOWER_RATE_LIMIT) - A_PULSE_WIDTH - A_REFRACTORY_PERIOD), msec)[A_CMP_DETECT == 0] % (60000msec/min) / (pulse/min) = msec / 1 pulse
    AAI.State_1 -> AAI.State_3 [order 1] : [A_CMP_DETECT == 1]
    AAI.State_3 -> AAI.State_1 : [after(A_REFRACTORY_PERIOD, msec)]
    AAI.State_2 -> AAI.State_3 : [after(A_PULSE_WIDTH, msec)]
  state VVI
    state State_1
      entry:
      FRONTEND_CTRL = 1
      %Charging C22
      ATR_PACE_CTRL = 0;
      VENT_PACE_CTRL = 0;
      PACING_REF_PWM = (V_PULSE_AMPLITUDE/5)*100;
      PACE_CHARGE_CTRL = 1;
      %Discharging Blocking Capacitor
      PACE_GND_CTRL = 1
      Z_ATR_CTRL = 0
      Z_VENT_CTRL = 0
      ATR_GND_CTRL = 0
      VENT_GND_CTRL = 1
    state State_2
      entry:
      %Ventricle Pacing
      PACE_CHARGE_CTRL = 0
      PACE_GND_CTRL = 1
      ATR_PACE_CTRL = 0
      ATR_GND_CTRL = 0
      Z_ATR_CTRL = 0
      Z_VENT_CTRL = 0
      VENT_GND_CTRL = 0
      VENT_PACE_CTRL = 1
    state State_3
      entry:
      %Charging C22
      ATR_PACE_CTRL = 0;
      VENT_PACE_CTRL = 0;
      PACING_REF_PWM = (V_PULSE_AMPLITUDE/5)*100;
      PACE_CHARGE_CTRL = 1;
      %Discharging Blocking Capacitor
      PACE_GND_CTRL = 1
      Z_ATR_CTRL = 0
      Z_VENT_CTRL = 0
      ATR_GND_CTRL = 0
      VENT_GND_CTRL = 1
    VVI.State_1 -> VVI.State_2 [order 2] : after(((60000/LOWER_RATE_LIMIT) - V_PULSE_WIDTH - V_REFRACTORY_PERIOD), msec)[V_CMP_DETECT == 0] % (60000msec/min) / (pulse/min) = msec / 1 pulse
    VVI.State_2 -> VVI.State_3 : [after(V_PULSE_WIDTH, msec)]
    VVI.State_1 -> VVI.State_3 [order 1] : [V_CMP_DETECT == 1]
    VVI.State_3 -> VVI.State_1 : [after(V_REFRACTORY_PERIOD, msec)]
  state AOOR
    state State_1
      entry:
      %Charging C22
      ATR_PACE_CTRL = 0;
      VENT_PACE_CTRL = 0;
      PACING_REF_PWM = (A_PULSE_AMPLITUDE/5)*100;
      PACE_CHARGE_CTRL = 1;
      %Discharging Blocking Capacitor
      PACE_GND_CTRL = 1
      Z_ATR_CTRL = 0
      Z_VENT_CTRL = 0
      ATR_GND_CTRL = 1
      VENT_GND_CTRL = 0
    state State_2
      entry:
      %Atrium Pacing
      PACE_CHARGE_CTRL = 0
      PACE_GND_CTRL = 1
      ATR_PACE_CTRL = 1
      ATR_GND_CTRL = 0
      Z_ATR_CTRL = 0
      Z_VENT_CTRL = 0
      VENT_GND_CTRL = 0
      VENT_PACE_CTRL = 0
    AOOR.State_1 -> AOOR.State_2 [order 1] : [after((30000/ADAPTIVE_RATE) - A_PULSE_WIDTH,msec)] % (60000msec/min) / (pulse/min) = msec / 1 pulse
    AOOR.State_2 -> AOOR.State_1 : [after(A_PULSE_WIDTH, msec)]
  state VOOR
    state State_1
      entry:
      %Charging C22
      ATR_PACE_CTRL = 0;
      VENT_PACE_CTRL = 0;
      PACING_REF_PWM = (V_PULSE_AMPLITUDE/5) * 100;
      PACE_CHARGE_CTRL = 1;
      %Discharging Blocking Capacitor
      PACE_GND_CTRL = 1
      Z_ATR_CTRL = 0
      Z_VENT_CTRL = 0
      ATR_GND_CTRL = 0
      VENT_GND_CTRL = 1
    state State_2
      entry:
      %Ventricle Pacing
      PACE_CHARGE_CTRL = 0
      PACE_GND_CTRL = 1
      ATR_PACE_CTRL = 0
      ATR_GND_CTRL = 0
      Z_ATR_CTRL = 0
      Z_VENT_CTRL = 0
      VENT_GND_CTRL = 0
      VENT_PACE_CTRL = 1
    VOOR.State_1 -> VOOR.State_2 [order 1] : [after((30000/ADAPTIVE_RATE) - V_PULSE_WIDTH,msec)] % (60000msec/min) / (pulse/min) = msec / 1 pulse
    VOOR.State_2 -> VOOR.State_1 : [after(V_PULSE_WIDTH, msec)]
  state AAIR
    state State_1
      entry:
      FRONTEND_CTRL = 1
      %Charging C22
      ATR_PACE_CTRL = 0;
      VENT_PACE_CTRL = 0;
      PACING_REF_PWM = (A_PULSE_AMPLITUDE/5)*100;
      PACE_CHARGE_CTRL = 1;
      %Discharging Blocking Capacitor
      PACE_GND_CTRL = 1
      Z_ATR_CTRL = 0
      Z_VENT_CTRL = 0
      ATR_GND_CTRL = 1
      VENT_GND_CTRL = 0
    state State_2
      entry:
      %Atrium Pacing
      PACE_CHARGE_CTRL = 0
      PACE_GND_CTRL = 1
      ATR_PACE_CTRL = 1
      ATR_GND_CTRL = 0
      Z_ATR_CTRL = 0
      Z_VENT_CTRL = 0
      VENT_GND_CTRL = 0
      VENT_PACE_CTRL = 0
    state State_3
      entry:
      %Charging C22
      ATR_PACE_CTRL = 0;
      VENT_PACE_CTRL = 0;
      PACING_REF_PWM = (A_PULSE_AMPLITUDE/5)*100;
      PACE_CHARGE_CTRL = 1;
      %Discharging Blocking Capacitor
      PACE_GND_CTRL = 1
      Z_ATR_CTRL = 0
      Z_VENT_CTRL = 0
      ATR_GND_CTRL = 1
      VENT_GND_CTRL = 0
    AAIR.State_1 -> AAIR.State_2 [order 2] : after(((30000/ADAPTIVE_RATE) - A_PULSE_WIDTH - A_REFRACTORY_PERIOD), msec)[A_CMP_DETECT == 0] % (60000msec/min) / (pulse/min) = msec / 1 pulse
    AAIR.State_1 -> AAIR.State_3 [order 1] : [A_CMP_DETECT == 1]
    AAIR.State_3 -> AAIR.State_1 : [after(A_REFRACTORY_PERIOD, msec)]
    AAIR.State_2 -> AAIR.State_3 : [after(A_PULSE_WIDTH, msec)]
  state VVIR
    state State_1
      entry:
      FRONTEND_CTRL = 1
      %Charging C22
      ATR_PACE_CTRL = 0;
      VENT_PACE_CTRL = 0;
      PACING_REF_PWM = (V_PULSE_AMPLITUDE/5)*100;
      PACE_CHARGE_CTRL = 1;
      %Discharging Blocking Capacitor
      PACE_GND_CTRL = 1
      Z_ATR_CTRL = 0
      Z_VENT_CTRL = 0
      ATR_GND_CTRL = 0
      VENT_GND_CTRL = 1
    state State_2
      entry:
      %Ventricle Pacing
      PACE_CHARGE_CTRL = 0
      PACE_GND_CTRL = 1
      ATR_PACE_CTRL = 0
      ATR_GND_CTRL = 0
      Z_ATR_CTRL = 0
      Z_VENT_CTRL = 0
      VENT_GND_CTRL = 0
      VENT_PACE_CTRL = 1
    state State_3
      entry:
      %Charging C22
      ATR_PACE_CTRL = 0;
      VENT_PACE_CTRL = 0;
      PACING_REF_PWM = (V_PULSE_AMPLITUDE/5)*100;
      PACE_CHARGE_CTRL = 1;
      %Discharging Blocking Capacitor
      PACE_GND_CTRL = 1
      Z_ATR_CTRL = 0
      Z_VENT_CTRL = 0
      ATR_GND_CTRL = 0
      VENT_GND_CTRL = 1
    VVIR.State_1 -> VVIR.State_2 [order 2] : after(((30000/ADAPTIVE_RATE) - V_PULSE_WIDTH - V_REFRACTORY_PERIOD), msec)[V_CMP_DETECT == 0] % (60000msec/min) / (pulse/min) = msec / 1 pulse
    VVIR.State_2 -> VVIR.State_3 : [after(V_PULSE_WIDTH, msec)]
    VVIR.State_1 -> VVIR.State_3 [order 1] : [V_CMP_DETECT == 1]
    VVIR.State_3 -> VVIR.State_1 : [after(V_REFRACTORY_PERIOD, msec)]
  state DDDR
    state State_5
      entry:
      FRONTEND_CTRL = 1
      %Charging C22
      ATR_PACE_CTRL = 0;
      VENT_PACE_CTRL = 0;
      PACING_REF_PWM = (A_PULSE_AMPLITUDE/5)*100;
      PACE_CHARGE_CTRL = 1;
      %Discharging Blocking Capacitor
      PACE_GND_CTRL = 1
      Z_ATR_CTRL = 0
      Z_VENT_CTRL = 0
      ATR_GND_CTRL = 1
      VENT_GND_CTRL = 1
    state State_4
      entry:
      %Atrium Pacing
      PACE_CHARGE_CTRL = 0
      PACE_GND_CTRL = 1
      ATR_PACE_CTRL = 1
      ATR_GND_CTRL = 0
      Z_ATR_CTRL = 0
      Z_VENT_CTRL = 0
      VENT_GND_CTRL = 0
      VENT_PACE_CTRL = 0
    state State_7
      entry:
      FRONTEND_CTRL = 1
      %Charging C22
      ATR_PACE_CTRL = 0;
      VENT_PACE_CTRL = 0;
      PACING_REF_PWM = (V_PULSE_AMPLITUDE/5)*100;
      PACE_CHARGE_CTRL = 1;
      %Discharging Blocking Capacitor
      PACE_GND_CTRL = 1
      Z_ATR_CTRL = 0
      Z_VENT_CTRL = 0
      ATR_GND_CTRL = 0
      VENT_GND_CTRL = 1
    state State_2
      entry:
      %Ventricle Pacing
      PACE_CHARGE_CTRL = 0
      PACE_GND_CTRL = 1
      ATR_PACE_CTRL = 0
      ATR_GND_CTRL = 0
      Z_ATR_CTRL = 0
      Z_VENT_CTRL = 0
      VENT_GND_CTRL = 0
      VENT_PACE_CTRL = 1
    state State_6
      entry:
      %Charging C22
      ATR_PACE_CTRL = 0;
      VENT_PACE_CTRL = 0;
      PACING_REF_PWM = (A_PULSE_AMPLITUDE/5)*100;
      PACE_CHARGE_CTRL = 1;
      %Discharging Blocking Capacitor
      PACE_GND_CTRL = 1
      Z_ATR_CTRL = 0
      Z_VENT_CTRL = 0
      ATR_GND_CTRL = 1
      VENT_GND_CTRL = 1
    State_4 -> State_7 [order 2] : [PUSHBUTTON ~= 1]
    State_7 -> DDDR.State_2 : after(FIXED_AV_DELAY,msec)
    State_5 -> State_4 [order 2] : after(((30000/ADAPTIVE_RATE) - A_PULSE_WIDTH - A_REFRACTORY_PERIOD), msec)[A_CMP_DETECT == 0] % (60000msec/min) / (pulse/min) = msec / 1 pulse
    State_5 -> State_6 [order 1] : [A_CMP_DETECT == 1]
    State_6 -> State_5 : [after(A_REFRACTORY_PERIOD, msec)]
    State_4 -> State_6 [order 1] : after(A_PULSE_WIDTH, msec)[PUSHBUTTON == 1]
    DDDR.State_2 -> State_6
  State_5 -> OFF [order 3] : [MODE ~= 9]
  (default) -> OFF
  AOOR.State_1 -> OFF [order 2] : [MODE ~= 5]
  VOOR.State_1 -> OFF [order 2] : [MODE ~= 6]
  AAIR.State_1 -> OFF [order 3] : [MODE ~= 7]
  VVIR.State_1 -> OFF [order 3] : [MODE ~= 8]
  OFF -> State_5 [order 9] : [MODE == 9]
  OFF -> AOOR.State_1 [order 5] : [MODE == 5]
  OFF -> VOOR.State_1 [order 6] : [MODE == 6]
  OFF -> AAIR.State_1 [order 7] : [MODE == 7]
  OFF -> VVIR.State_1 [order 8] : [MODE == 8]
  OFF -> AAI.State_1 [order 4] : [MODE == 3]
  AAI.State_1 -> OFF [order 3] : [MODE ~= 3]
  VVI.State_1 -> OFF [order 3] : [MODE ~= 4]
  OFF -> VVI.State_1 [order 3] : [MODE == 4]
  VOO.State_1 -> OFF [order 2] : [MODE ~= 2]
  OFF -> VOO.State_1 [order 2] : [MODE == 2]
  AOO.State_1 -> OFF [order 1] : [MODE ~= 1]
  OFF -> AOO.State_1 [order 1] : [MODE == 1]
  data: MODE input; LOWER_RATE_LIMIT input; Z_ATR_CTRL output; PACING_REF_PWM output; ATR_PACE_CTRL output; PACE_GND_CTRL output; ATR_GND_CTRL output; PACE_CHARGE_CTRL output; VENT_PACE_CTRL output; VENT_GND_CTRL output; Z_VENT_CTRL output; FRONTEND_CTRL output; ADAPTIVE_RATE input; A_PULSE_AMPLITUDE input; V_PULSE_AMPLITUDE input; A_PULSE_WIDTH input; V_PULSE_WIDTH input; V_REFRACTORY_PERIOD input; A_REFRACTORY_PERIOD input; V_CMP_DETECT input; A_CMP_DETECT input; PUSHBUTTON input; FIXED_AV_DELAY input

== matlab function Pacemaker_Simulink/Subsystem/Subsystem/MATLAB Function1 ==
  data: ACTIVITY_LEVEL input; DESIRED_PACING_RATE output; ACTIVITY_THRESHOLD input; RESPONSE_FACTOR input; LOWER_RATE_LIMIT input; MAXIMUM_SENSOR_RATE input
function DESIRED_PACING_RATE = fcn(ACTIVITY_LEVEL, ACTIVITY_THRESHOLD, RESPONSE_FACTOR, LOWER_RATE_LIMIT, MAXIMUM_SENSOR_RATE)
    if ACTIVITY_LEVEL >= ACTIVITY_THRESHOLD
        slope = (MAXIMUM_SENSOR_RATE-LOWER_RATE_LIMIT)/((ACTIVITY_THRESHOLD + (((1.6-ACTIVITY_THRESHOLD)/16)*(16-(RESPONSE_FACTOR-1)))) - ACTIVITY_THRESHOLD);
        b = LOWER_RATE_LIMIT - (slope*(ACTIVITY_THRESHOLD));
        if(slope*ACTIVITY_LEVEL + b > MAXIMUM_SENSOR_RATE)
            DESIRED_PACING_RATE = MAXIMUM_SENSOR_RATE;
        else
            DESIRED_PACING_RATE = slope*ACTIVITY_LEVEL + b;
        end
    else
        DESIRED_PACING_RATE = LOWER_RATE_LIMIT;
    end
end

== matlab function Pacemaker_Simulink/Subsystem/MATLAB Function ==
  data: MODE input; y output
function y = fcn(MODE)
    if MODE > 4
        y = 1;
    else
        y = 0;
    end
